simulink model "Q1"  (R2021a)
settings: Solver=VariableStepAuto  StartTime=0.0  StopTime=100  RelTol=1e-3
settings Model: Creator=viral  LastModifiedBy=viral

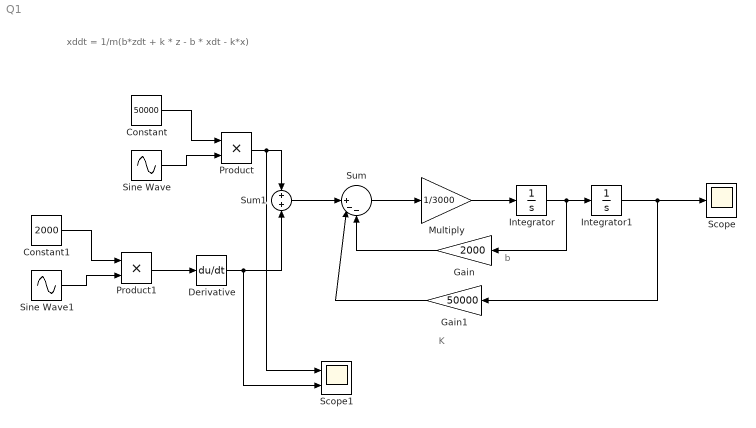
== system Q1 ==
  note: K
  note: xddt = 1/m(b*zdt + k * z - b * xdt - k*x)
  note: b
  Constant : Constant  Value=50000
  Constant1 : Constant  Value=2000
  Derivative : Derivative
  Gain : Gain  Gain=2000
  Gain1 : Gain  Gain=50000
  Integrator : Integrator
  Integrator1 : Integrator
  Multiply : Gain  Gain=1/3000
  Product : Product
  Product1 : Product
  Scope : Scope
  Scope1 : Scope  NumInputPorts=2
  Sine Wave : Sin  Amplitude=0.01  Frequency=3.5  SampleTime=0
  Sine Wave1 : Sin  Amplitude=0.01  Frequency=3.5  SampleTime=0
  Sum : Sum  Inputs=||+--
  Sum1 : Sum  Inputs=+|+
  wires:
  Integrator/1 -> Gain/1, Integrator1/1
  Integrator1/1 -> Gain1/1, Scope/1
  Gain/1 -> Sum/3
  Gain1/1 -> Sum/2
  Multiply/1 -> Integrator/1
  Sine Wave/1 -> Product/2
  Constant/1 -> Product/1
  Product/1 -> Scope1/1, Sum1/1
  Sine Wave1/1 -> Product1/2
  Constant1/1 -> Product1/1
  Product1/1 -> Derivative/1
  Derivative/1 -> Scope1/2, Sum1/2
  Sum1/1 -> Sum/1
  Sum/1 -> Multiply/1
